simulink model "SimplePhoenixModel_2016"  (R2016a)
settings: Solver=VariableStepAuto  SolverMode=SingleTasking  StartTime=0.0  StopTime=100  RelTol=1e-3
libraries: simulink x1
settings Model: Creator=GusBus  LastModifiedBy=GusBus
settings DebuggingCC: SFUnexpectedBacktrackingDiag=error  SFNoUnconditionalDefaultTransitionDiag=error
settings GRTTargetCC: TargetLangStandard=C99 (ISO)  GeneratePreprocessorConditionals=Use local settings
settings ConfigComp: CovMetricSettings=dwe  CovHtmlReporting=off  CovSaveCumulativeToWorkspaceVar=off  CovSaveSingleToWorkspaceVar=off  CovExternalEMLEnable=on

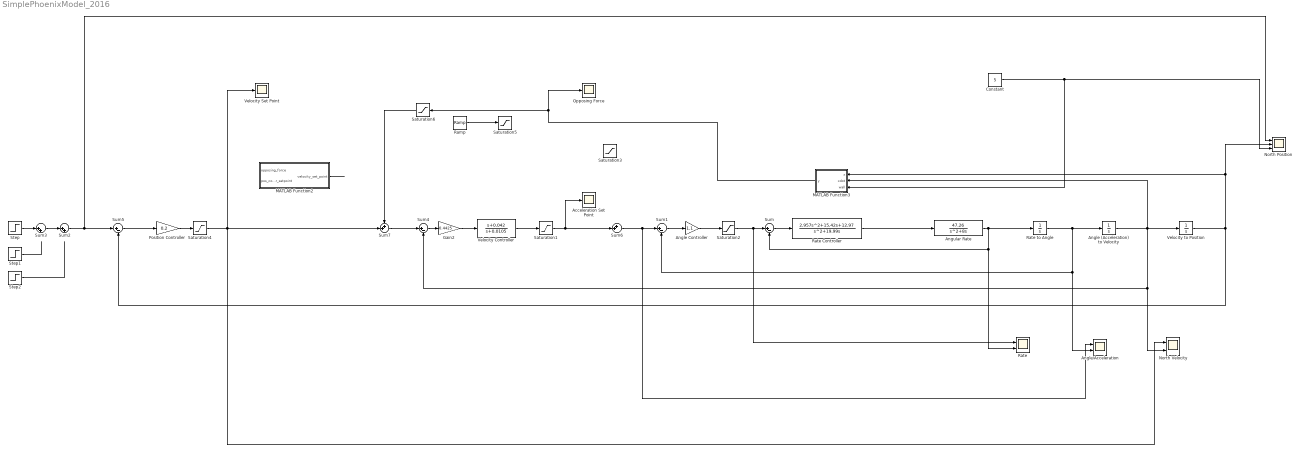
== system SimplePhoenixModel_2016 ==
  Acceleration Set Point : Scope
  Angle (Acceleration) to Velocity : Integrator
  Angle Controller : Gain  Gain=1.1
  Angle/Acceleration : Scope  NumInputPorts=2
  Angular Rate : TransferFcn  Numerator=[47.26]  Denominator=[1 8 0]
  Constant : Constant  Value=5
  Gain2 : Gain  Gain=0.4425
  MATLAB Function2 : MATLAB Function  TreatAsAtomicUnit=on
  MATLAB Function3 : MATLAB Function  TreatAsAtomicUnit=on
  North Position : Scope  NumInputPorts=3
  North Velocity : Scope  NumInputPorts=2
  Opposing Force : Scope
  Position Controller : Gain  Gain=0.2
  Ramp : simulink/Sources/Ramp  slope=-1  start=0  X0=0
  Rate : Scope  NumInputPorts=2
  Rate Controller : TransferFcn  Numerator=[2.957 15.42 12.97]  Denominator=[1 19.99 0]
  Rate to Angle : Integrator
  Saturation1 : Saturate  UpperLimit=4  LowerLimit=-4
  Saturation2 : Saturate  UpperLimit=5  LowerLimit=-5
  Saturation3 : Saturate  UpperLimit=3  LowerLimit=-3
  Saturation4 : Saturate  UpperLimit=1  LowerLimit=-1
  Saturation5 : Saturate  UpperLimit=0  LowerLimit=-1
  Saturation6 : Saturate  UpperLimit=3  LowerLimit=-3
  Step : Step  After=10  SampleTime=0
  Step1 : Step  Time=20  After=6  SampleTime=0
  Step2 : Step  Time=50  After=-8  SampleTime=0
  Sum{,1,4..5} (4 alike) : Sum  Inputs=|+-
  Sum2 : Sum  Inputs=|++
  Sum3 : Sum  Inputs=|++
  Sum6 : Sum  Inputs=++|
  Sum7 : Sum  Inputs=++|
  Velocity Controller : TransferFcn  Numerator=[1 0.042]  Denominator=[1 0.0105]
  Velocity Set Point : Scope
  Velocity to Position : Integrator
  wires:
  Step/1 -> Sum3/1
  Step1/1 -> ?
  Rate to Angle/1 -> Angle (Acceleration) to Velocity/1, Angle/Acceleration/2, Sum1/2
  Step2/1 -> ?
  Sum/1 -> Rate Controller/1
  Angular Rate/1 -> Rate/2, Sum/2, Rate to Angle/1
  Angle (Acceleration) to Velocity/1 -> MATLAB Function3/2(xdot), Velocity to Position/1, North Velocity/2, Sum4/2
  Sum1/1 -> Angle Controller/1
  Sum3/1 -> Sum2/1
  Gain2/1 -> Velocity Controller/1
  Sum5/1 -> Position Controller/1
  Velocity to Position/1 -> MATLAB Function3/1(x), North Position/2, Sum5/2
  Sum2/1 -> Sum5/1, North Position/1
  Sum6/1 -> Angle/Acceleration/1, Sum1/1
  Sum4/1 -> Gain2/1
  Rate Controller/1 -> Angular Rate/1
  Ramp/1 -> Saturation5/1
  Sum7/1 -> Sum4/1
  Constant/1 -> MATLAB Function3/3(wall), North Position/3
  Position Controller/1 -> Saturation4/1
  Velocity Controller/1 -> Saturation1/1
  Angle Controller/1 -> Saturation2/1
  Saturation4/1 -> Sum7/2, North Velocity/1, Velocity Set Point/1
  MATLAB Function3/1(y) -> Saturation6/1, Opposing Force/1
  MATLAB Function2/1(velocity_set_point) -> ?
  Saturation1/1 -> Acceleration Set Point/1, Sum6/2
  Saturation2/1 -> Rate/1, Sum/1
  Saturation6/1 -> Sum7/1

== matlab function SimplePhoenixModel_2016/MATLAB Function2 ==
  data: opposing_force input; velocity_set_point output; pos_controller_setpoint input
function velocity_set_point = fcn(opposing_force, pos_controller_setpoint)

%if the opposing force is bigger than some hysteris around 0 and the
%opposing force and velocity setpoint are not in the same direction then
%set to opposing force

% if abs(opposing_force) >= 0.001
%     velocity_set_point = opposing_force;
% else
%     velocity_set_point = pos_controller_setpoint;
% end

if abs(opposing_force) >= 0.001
    if pos_controller_setpoint > 0 && opposing_force > 0
        velocity_set_point = pos_controller_setpoint;
    elseif pos_controller_setpoint < 0 && opposing_force < 0
        velocity_set_point = pos_controller_setpoint
    else
        velocity_set_point = opposing_force;
    end
else
    velocity_set_point = pos_controller_setpoint;
end

== matlab function SimplePhoenixModel_2016/MATLAB Function3 ==
  data: x input; y output; xdot input; wall input
function y = fcn(x,xdot,wall)

%Wall at 5m
sensor_max_distance = 2.5;
sensor_direction = 0;
distance_to_wall = wall-x;

% % Coefficinets used in summing option
% ks = 1;
% kd = 5;

% % Coefficients used in modified min max option
ks = 0.5;
kd = 2.2;


%If we are further away from the wall than the sensor can read, set sensor
%reading to 0 (disable spring) and xdot to zero (disable damping)
%Otherwise calculate the sensor reading by subtracting it from the distance
%to the wall

% at 2m from the wall distance from wall = 2 sensor reading = 0
% at 1m from wall sensor reading = 1
% at 0m from the wall sensor reading = max = 2

if abs(distance_to_wall) > sensor_max_distance
    sensor_reading = 0;
    xdot = 0;
elseif distance_to_wall < 0
    sensor_reading = -sensor_max_distance - distance_to_wall;
    sensor_direction = -1;
else     
    sensor_reading = sensor_max_distance - distance_to_wall;
    sensor_direction = 1;
end

y = sensor_direction*ks*(sensor_reading^2) + kd*xdot;

%However we would like the force to oppose the motion
y = -y;
